simulink library "csu_tpl_thruster_propellant_mtv_lib"  (R2014b)
settings: Solver=ode45  StartTime=0.0  StopTime=10.0  RelTol=1e-3
values from neighbouring files (symbols this model uses):
  tpl_coarse_acs_thrust_to_isp = [ ... (first row only)    [csu_tpl_thruster_propellant_mtv_prep.m]
libraries: util_info_lib x1
settings Model: Creator=Nilesh  LastModifiedBy=mstewart

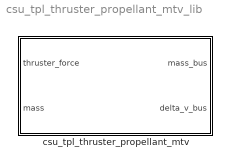
== system csu_tpl_thruster_propellant_mtv_lib ==
  csu_tpl_thruster_propellant_mtv : Subsystem

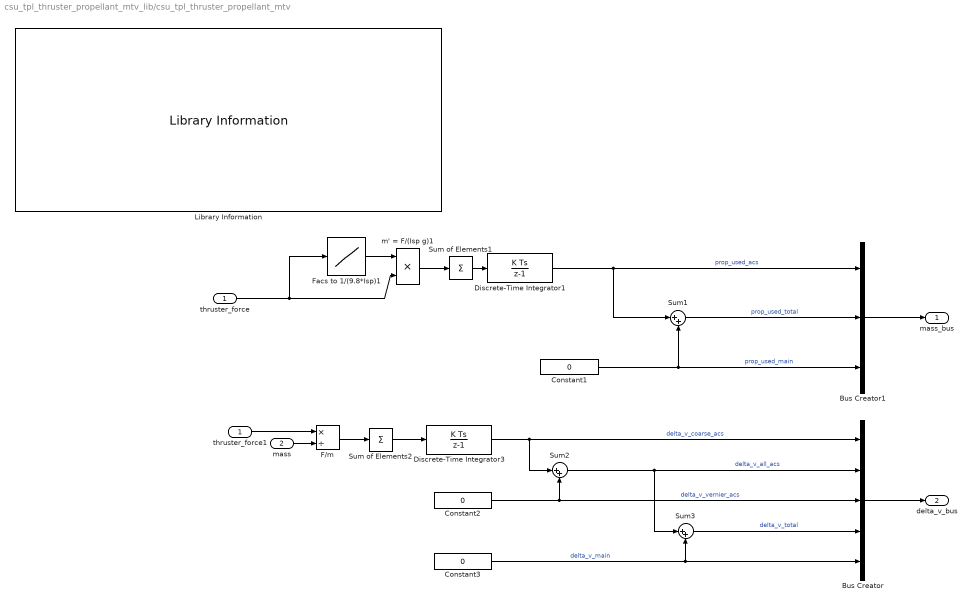
== system csu_tpl_thruster_propellant_mtv_lib/csu_tpl_thruster_propellant_mtv ==
  thruster_force : Inport
  mass : Inport  Port=2
  Bus Creator : BusCreator  Inputs=5
  Bus Creator1 : BusCreator  Inputs=3
  Constant1 : Constant  Value=0  OutDataTypeStr=double
  Constant2 : Constant  Value=0  OutDataTypeStr=double
  Constant3 : Constant  Value=0  OutDataTypeStr=double
  Discrete-Time Integrator1 : DiscreteIntegrator  gainval=1  SampleTime=-1
  Discrete-Time Integrator3 : DiscreteIntegrator  gainval=1  SampleTime=-1
  F/m : Product  Inputs=*/
  Facs to 1/(9.8*Isp)1 : Lookup  InputValues=tpl_coarse_acs_thrust_to_isp(:,1)  Table=1./(9.8*tpl_coarse_acs_thrust_to_isp(:,2))  LookUpMeth=Interpolation-Use End Values
  Library Information : util_info_lib/Library Information  owner='escrane'
  Sum of Elements1 : Sum  Inputs=+
  Sum of Elements2 : Sum  Inputs=+
  Sum1 : Sum  Inputs=|++
  Sum2 : Sum  Inputs=|++
  Sum3 : Sum  Inputs=|++
  m' = F/(Isp g)1 : Product  RndMeth=Zero
  thruster_force1 : InportShadow
  mass_bus : Outport
  delta_v_bus : Outport  Port=2
  wires:
  thruster_force1/1 -> F/m/1
  Bus Creator1/1 -> mass_bus/1
  Bus Creator/1 -> delta_v_bus/1
  Constant3/1 -> Bus Creator/5, Sum3/2  "delta_v_main"
  Sum3/1 -> Bus Creator/4  "delta_v_total"
  Sum of Elements2/1 -> Discrete-Time Integrator3/1
  F/m/1 -> Sum of Elements2/1
  mass/1 -> F/m/2
  Constant1/1 -> Bus Creator1/3, Sum1/2  "prop_used_main"
  Sum of Elements1/1 -> Discrete-Time Integrator1/1
  thruster_force/1 -> m' = F/(Isp g)1/2, Facs to 1/(9.8*Isp)1/1
  Facs to 1/(9.8*Isp)1/1 -> m' = F/(Isp g)1/1
  m' = F/(Isp g)1/1 -> Sum of Elements1/1
  Sum1/1 -> Bus Creator1/2  "prop_used_total"
  Discrete-Time Integrator1/1 -> Bus Creator1/1, Sum1/1  "prop_used_acs"
  Constant2/1 -> Bus Creator/3, Sum2/2  "delta_v_vernier_acs"
  Discrete-Time Integrator3/1 -> Bus Creator/1, Sum2/1  "delta_v_coarse_acs"
  Sum2/1 -> Bus Creator/2, Sum3/1  "delta_v_all_acs"
